simulink model "controlador2015"  (R2015a)
settings: Solver=ode1  SolverMode=SingleTasking  StartTime=0.0  StopTime=Tsimu  FixedStep=h  RelTol=1e-3
values from neighbouring files (symbols this model uses):
  A = [(rgo*Cwro2 - Cwpg2) (rgo*Cwro3 - Cwpg3); (Cwro2 - Cwpo2) (Cwro3 - Cwpo3)]    [init.m]
  B = [1 0]'    [init.m]
  C = g/Aw*[1 1]    [init.m]
  h = 0.1    [init.m]
  K0 = place(A, B, [-5 -6])    [init.m]
  N0 = 1/(C*inv(-1*(A - B*K0))*B)    [init.m]
  r0 = 1    [init.m]
  Tsimu = 100e3    (= 100000)    [init.m]
  x0 = [0 0]'    [init.m]
libraries: simulink x1
settings Model: CovMetricSettings=dwe  CovHtmlReporting=off  covSaveCumulativeToWorkspaceVar=off  CovSaveSingleToWorkspaceVar=off  CovExternalEMLEnable=on  Creator=Raposo  LastModifiedBy=raposo
settings DataIOCC: LimitDataPoints=off  SaveFormat=Dataset
settings DebuggingCC: SFUnexpectedBacktrackingDiag=error  SFNoUnconditionalDefaultTransitionDiag=error
settings HardwareCC: ProdBitPerPointer=64  ProdLargestAtomicFloat=Float  ProdIntDivRoundTo=Zero  ProdEndianess=LittleEndian  ProdHWDeviceType=Specified
settings ModelReferenceCC: PropagateSignalLabelsOutOfModel=on
settings GRTTargetCC: TargetLangStandard=C99 (ISO)  GeneratePreprocessorConditionals=Use local settings

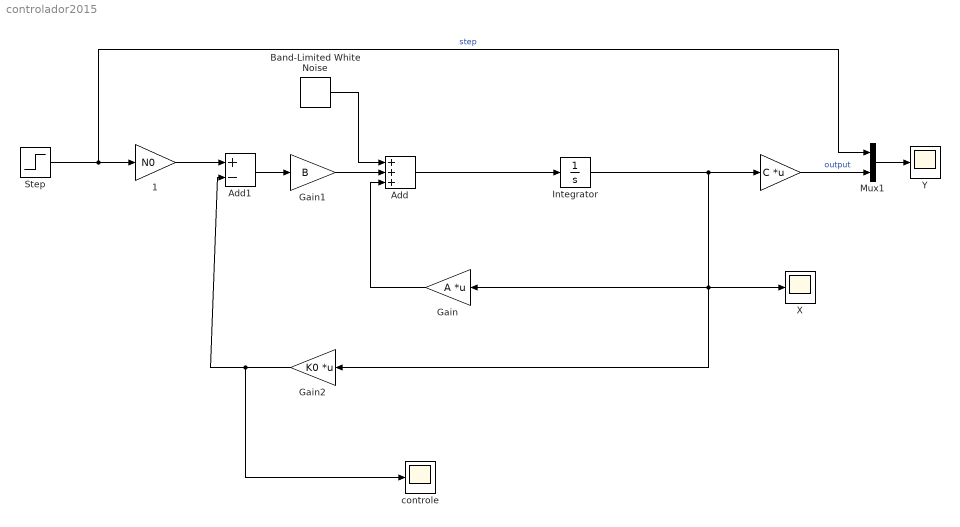
== system controlador2015 ==
  " " : Gain  Gain=C  Multiplication=Matrix(K*u)
  " 1" : Gain  Gain=N0
  Add : Sum  Inputs=+++
  Add1 : Sum  Inputs=+-
  Band-Limited White Noise : simulink/Sources/Band-Limited White Noise  Cov=[0.00000001]*0  Ts=h  seed=[23341]
  Gain : Gain  Gain=A  Multiplication=Matrix(K*u)
  Gain1 : Gain  Gain=B
  Gain2 : Gain  Gain=K0  Multiplication=Matrix(K*u)
  Integrator : Integrator  InitialCondition=x0
  Mux1 : Mux  Inputs=2
  Step : Step  Time=Tsimu/2  After=r0  SampleTime=h
  X : Scope
      settings: TimeRange=auto  ShowLegends=on  MaxDataPoints=5000  SaveToWorkspace=off  SaveName=ScopeData  YMin=-19.65069  YMax=2.21041  SampleTime=-1
  Y : Scope
      settings: TimeRange=auto  ShowLegends=on  MaxDataPoints=5000  SaveToWorkspace=off  SaveName=ScopeData2  YMin=-949.60026  YMax=106.62225  SampleInput=on  SampleTime=h
  controle : Scope
      settings: TimeRange=auto  ShowLegends=on  MaxDataPoints=5000  SaveToWorkspace=off  YMin=-0.74681  YMax=0.12101  SampleTime=-1
  wires:
  Band-Limited White Noise/1 -> Add/1
  Gain/1 -> Add/3
  Step/1 -> " 1"/1, Mux1/1  "step"
  Mux1/1 -> Y/1
  " "/1 -> Mux1/2  "output"
  Add1/1 -> Gain1/1
  Gain1/1 -> Add/2
  Add/1 -> Integrator/1
  Integrator/1 -> Gain2/1, X/1, Gain/1, " "/1
  Gain2/1 -> controle/1, Add1/2
  " 1"/1 -> Add1/1
